simulink model "ChimeIndicatorOutput"  (R2018b)
settings: Solver=FixedStepDiscrete  StartTime=0.0  StopTime=10.0  FixedStep=0.01  RelTol=1e-3
undefined symbols (not defined in the file or in its folder): f, h, IfVeSMSeStNumConfig, KeSMSbMdChime1Enable_Val, KeSMSbSRSPosNumConfig_Val, KeSMSuChmReqDurmTm_Val, KeSMSuChmReqIntlTm_Val, KeSMSwModeChimeReqTm_Val, KeSMSwSRSActiveValidTm_Val, SRSIndicatorStat1
libraries: MSMLib x27
(part 1 of 2)
settings Model: Creator=su3dcu  LastModifiedBy=su3dcu
settings DataIOCC: SaveFormat=StructureWithTime
settings OptimizationCC: DefaultParameterBehavior=Inlined  EnhancedBackFolding=on  PassReuseOutputArgsAs=Individual arguments  ZeroExternalMemoryAtStartup=off  ZeroInternalMemoryAtStartup=off  OptimizeBlockOrder=speed  DifferentSizesBufferReuse=on  OptimizationCustomize=off
settings DebuggingCC: ParameterTunabilityLossMsg=error
settings HardwareCC: ProdBitPerPointer=32  ProdBitPerSizeT=32  ProdBitPerPtrDiffT=32  ProdLargestAtomicFloat=None  ProdWordSize=32  ProdHWDeviceType=Renesas->RH850
settings ModelReferenceCC: ModelReferenceNumInstancesAllowed=Single
settings SFSimCC: MATLABDynamicMemAlloc=off
settings RTWCC: SystemTargetFile=autosar.tlc  GenCodeOnly=on  TemplateMakefile=ert_default_tmf  Description=AUTOSAR  GenerateReport=on  IncludeHyperlinkInReport=on  LaunchReport=on  GenerateTraceInfo=on  GenerateTraceReport=on  GenerateTraceReportSl=on  GenerateTraceReportSf=on  GenerateTraceReportEml=on
settings CodeAppCC: ForceParamTrailComments=on  IgnoreCustomStorageClasses=off  OperatorAnnotations=on  SimulinkDataObjDesc=on  SFDataObjDesc=on  InsertBlockDesc=on
settings STFCustomTargetCC: TargetLangStandard=C99 (ISO)  MultiwordLength=256  ParMdlRefBuildCompliant=on  CompOptLevelCompliant=on  IncludeMdlTerminateFcn=off  CombineOutputUpdateFcns=on  SuppressErrorStatus=on  ERTCustomFileBanners=on  SupportNonFinite=off  SupportComplex=off  SupportContinuousTime=off  SupportNonInlinedSFcns=off  RemoveResetFunc=on  MATLABClassNameForMDSCustomization=Simulink.SoftwareTarget.ERTCustomization  AutosarCompliant=on  UseToolchainInfoCompliant=on  LookupTableObjectStructAxisOrder=2,1,3,4,...  LUTObjectStructOrderEvenSpacing=Size,Table,Breakpoints  SystemTargetFile=autosar.tlc
settings ERTTargetCC: TargetLangStandard=C99 (ISO)  ConcurrentExecutionCompliant=off  IncludeMdlTerminateFcn=off  SuppressErrorStatus=on  SupportNonFinite=off  SupportComplex=off  ModelStepFunctionPrototypeControlCompliant=off  CPPClassGenCompliant=off  AutosarCompliant=on  LookupTableObjectStructAxisOrder=2,1,3,4,...  LUTObjectStructOrderEvenSpacing=Size,Table,Breakpoints  InlinedParameterPlacement=NonHierarchical  ERTCustomFileTemplate=example_file_process.tlc  ERTFilePackagingFormat=Compact

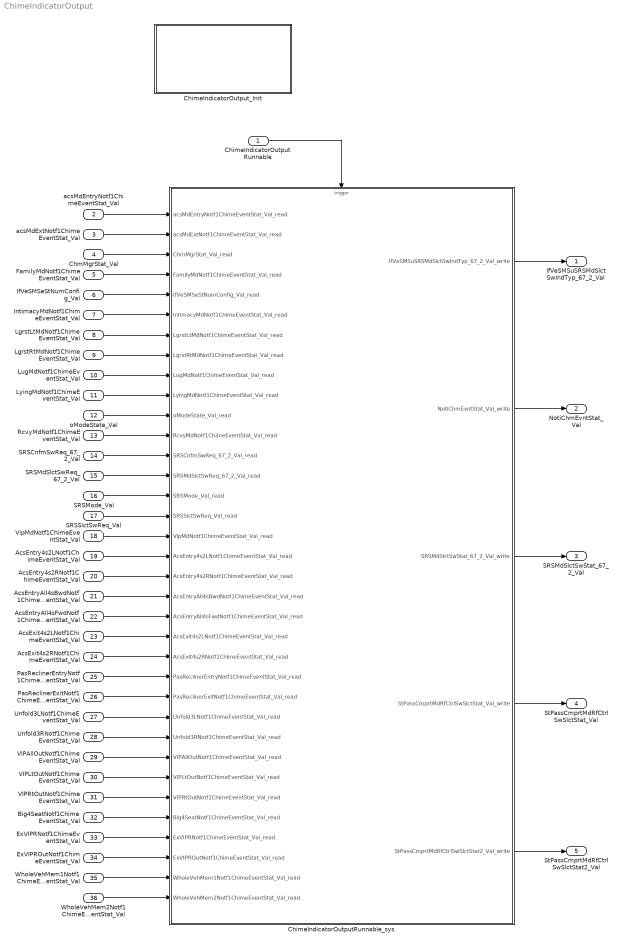
== system ChimeIndicatorOutput ==
  ChimeIndicatorOutputRunnable : Inport  SampleTime=0.01  OutputFunctionCall=on
  acsMdEntryNotf1ChimeEventStat_Val : Inport  Port=2  OutDataTypeStr=boolean  PortDimensions=1
  acsMdExtNotf1ChimeEventStat_Val : Inport  Port=3  OutDataTypeStr=boolean  PortDimensions=1
  ChmMgrStat_Val : Inport  Port=4  OutDataTypeStr=uint16  PortDimensions=1
  FamilyMdNotf1ChimeEventStat_Val : Inport  Port=5  OutDataTypeStr=boolean  PortDimensions=1
  IfVeSMSeStNumConfig_Val : Inport  Port=6  OutDataTypeStr=Enum: IfVeSMSeStNumConfig  PortDimensions=1
  IntimacyMdNotf1ChimeEventStat_Val : Inport  Port=7  OutDataTypeStr=boolean  PortDimensions=1
  LgrstLtMdNotf1ChimeEventStat_Val : Inport  Port=8  OutDataTypeStr=boolean  PortDimensions=1
  LgrstRtMdNotf1ChimeEventStat_Val : Inport  Port=9  OutDataTypeStr=boolean  PortDimensions=1
  LugMdNotf1ChimeEventStat_Val : Inport  Port=10  OutDataTypeStr=boolean  PortDimensions=1
  LyingMdNotf1ChimeEventStat_Val : Inport  Port=11  OutDataTypeStr=boolean  PortDimensions=1
  oModeState_Val : Inport  Port=12  OutDataTypeStr=Enum: MdTp1  PortDimensions=1
  RcvyMdNotf1ChimeEventStat_Val : Inport  Port=13  OutDataTypeStr=boolean  PortDimensions=1
  SRSCnfmSwReq_67_2_Val : Inport  Port=14  OutDataTypeStr=boolean  PortDimensions=1
  SRSMdSlctSwReq_67_2_Val : Inport  Port=15  OutDataTypeStr=Enum: SRSSlctSwStat1  PortDimensions=1
  SRSMode_Val : Inport  Port=16  OutDataTypeStr=Enum: SRSCurMode1  PortDimensions=1
  SRSSlctSwReq_Val : Inport  Port=17  OutDataTypeStr=Enum: SRSMode1  PortDimensions=1
  VipMdNotf1ChimeEventStat_Val : Inport  Port=18  OutDataTypeStr=boolean  PortDimensions=1
  AcsEntry4s2LNotf1ChimeEventStat_Val : Inport  Port=19  OutDataTypeStr=boolean  PortDimensions=1
  AcsEntry4s2RNotf1ChimeEventStat_Val : Inport  Port=20  OutDataTypeStr=boolean  PortDimensions=1
  AcsEntryAll4sBwdNotf1ChimeEventStat_Val : Inport  Port=21  OutDataTypeStr=boolean  PortDimensions=1
  AcsEntryAll4sFwdNotf1ChimeEventStat_Val : Inport  Port=22  OutDataTypeStr=boolean  PortDimensions=1
  AcsExit4s2LNotf1ChimeEventStat_Val : Inport  Port=23  OutDataTypeStr=boolean  PortDimensions=1
  AcsExit4s2RNotf1ChimeEventStat_Val : Inport  Port=24  OutDataTypeStr=boolean  PortDimensions=1
  PasReclinerEntryNotf1ChimeEventStat_Val : Inport  Port=25  OutDataTypeStr=boolean  PortDimensions=1
  PasReclinerExitNotf1ChimeEventStat_Val : Inport  Port=26  OutDataTypeStr=boolean  PortDimensions=1
  Unfold3LNotf1ChimeEventStat_Val : Inport  Port=27  OutDataTypeStr=boolean  PortDimensions=1
  Unfold3RNotf1ChimeEventStat_Val : Inport  Port=28  OutDataTypeStr=boolean  PortDimensions=1
  VIPAllOutNotf1ChimeEventStat_Val : Inport  Port=29  OutDataTypeStr=boolean  PortDimensions=1
  VIPLtOutNotf1ChimeEventStat_Val : Inport  Port=30  OutDataTypeStr=boolean  PortDimensions=1
  VIPRtOutNotf1ChimeEventStat_Val : Inport  Port=31  OutDataTypeStr=boolean  PortDimensions=1
  Big4SeatNotf1ChimeEventStat_Val : Inport  Port=32  OutDataTypeStr=boolean  PortDimensions=1
  ExVIPRNotf1ChimeEventStat_Val : Inport  Port=33  OutDataTypeStr=boolean  PortDimensions=1
  ExVIPROutNotf1ChimeEventStat_Val : Inport  Port=34  OutDataTypeStr=boolean  PortDimensions=1
  WholeVehMem1Notf1ChimeEventStat_Val : Inport  Port=35  OutDataTypeStr=boolean  PortDimensions=1
  WholeVehMem2Notf1ChimeEventStat_Val : Inport  Port=36  OutDataTypeStr=boolean  PortDimensions=1
  ChimeIndicatorOutputRunnable_sys : Subsystem
  ChimeIndicatorOutput_Init : Subsystem
  IfVeSMSuSRSMdSlctSwIndTyp_67_2_Val : Outport  OutDataTypeStr=Enum: SRSSlctSwIndTyp  PortDimensions=1
  NotiChmEvntStat_Val : Outport  Port=2  OutDataTypeStr=Enum: EventSts1  PortDimensions=1
  SRSMdSlctSwStat_67_2_Val : Outport  Port=3  OutDataTypeStr=Enum: SRSIndicatorStat  PortDimensions=1
  StPassCmprtMdRfCtrlSwSlctStat_Val : Outport  Port=4  OutDataTypeStr=Enum: CmprtMdRfCtrlSwSlctStat1  PortDimensions=1
  StPassCmprtMdRfCtrlSwSlctStat2_Val : Outport  Port=5  OutDataTypeStr=Enum: CmprtMdRfCtrlSwSlctStat2  PortDimensions=1
  wires:
  acsMdEntryNotf1ChimeEventStat_Val/1 -> ChimeIndicatorOutputRunnable_sys/1(acsMdEntryNotf1ChimeEventStat_Val_read)
  acsMdExtNotf1ChimeEventStat_Val/1 -> ChimeIndicatorOutputRunnable_sys/2(acsMdExtNotf1ChimeEventStat_Val_read)
  ChmMgrStat_Val/1 -> ChimeIndicatorOutputRunnable_sys/3(ChmMgrStat_Val_read)
  FamilyMdNotf1ChimeEventStat_Val/1 -> ChimeIndicatorOutputRunnable_sys/4(FamilyMdNotf1ChimeEventStat_Val_read)
  IfVeSMSeStNumConfig_Val/1 -> ChimeIndicatorOutputRunnable_sys/5(IfVeSMSeStNumConfig_Val_read)
  IntimacyMdNotf1ChimeEventStat_Val/1 -> ChimeIndicatorOutputRunnable_sys/6(IntimacyMdNotf1ChimeEventStat_Val_read)
  LgrstLtMdNotf1ChimeEventStat_Val/1 -> ChimeIndicatorOutputRunnable_sys/7(LgrstLtMdNotf1ChimeEventStat_Val_read)
  LgrstRtMdNotf1ChimeEventStat_Val/1 -> ChimeIndicatorOutputRunnable_sys/8(LgrstRtMdNotf1ChimeEventStat_Val_read)
  LugMdNotf1ChimeEventStat_Val/1 -> ChimeIndicatorOutputRunnable_sys/9(LugMdNotf1ChimeEventStat_Val_read)
  LyingMdNotf1ChimeEventStat_Val/1 -> ChimeIndicatorOutputRunnable_sys/10(LyingMdNotf1ChimeEventStat_Val_read)
  oModeState_Val/1 -> ChimeIndicatorOutputRunnable_sys/11(oModeState_Val_read)
  RcvyMdNotf1ChimeEventStat_Val/1 -> ChimeIndicatorOutputRunnable_sys/12(RcvyMdNotf1ChimeEventStat_Val_read)
  SRSCnfmSwReq_67_2_Val/1 -> ChimeIndicatorOutputRunnable_sys/13(SRSCnfmSwReq_67_2_Val_read)
  SRSMdSlctSwReq_67_2_Val/1 -> ChimeIndicatorOutputRunnable_sys/14(SRSMdSlctSwReq_67_2_Val_read)
  SRSMode_Val/1 -> ChimeIndicatorOutputRunnable_sys/15(SRSMode_Val_read)
  SRSSlctSwReq_Val/1 -> ChimeIndicatorOutputRunnable_sys/16(SRSSlctSwReq_Val_read)
  VipMdNotf1ChimeEventStat_Val/1 -> ChimeIndicatorOutputRunnable_sys/17(VipMdNotf1ChimeEventStat_Val_read)
  ChimeIndicatorOutputRunnable_sys/1(IfVeSMSuSRSMdSlctSwIndTyp_67_2_Val_write) -> IfVeSMSuSRSMdSlctSwIndTyp_67_2_Val/1
  ChimeIndicatorOutputRunnable_sys/2(NotiChmEvntStat_Val_write) -> NotiChmEvntStat_Val/1
  ChimeIndicatorOutputRunnable_sys/3(SRSMdSlctSwStat_67_2_Val_write) -> SRSMdSlctSwStat_67_2_Val/1
  ChimeIndicatorOutputRunnable_sys/4(StPassCmprtMdRfCtrlSwSlctStat_Val_write) -> StPassCmprtMdRfCtrlSwSlctStat_Val/1
  ChimeIndicatorOutputRunnable_sys/5(StPassCmprtMdRfCtrlSwSlctStat2_Val_write) -> StPassCmprtMdRfCtrlSwSlctStat2_Val/1
  ChimeIndicatorOutputRunnable/1 -> ChimeIndicatorOutputRunnable_sys/Trigger
  AcsEntry4s2LNotf1ChimeEventStat_Val/1 -> ChimeIndicatorOutputRunnable_sys/18(AcsEntry4s2LNotf1ChimeEventStat_Val_read)
  AcsEntry4s2RNotf1ChimeEventStat_Val/1 -> ChimeIndicatorOutputRunnable_sys/19(AcsEntry4s2RNotf1ChimeEventStat_Val_read)
  AcsEntryAll4sBwdNotf1ChimeEventStat_Val/1 -> ChimeIndicatorOutputRunnable_sys/20(AcsEntryAll4sBwdNotf1ChimeEventStat_Val_read)
  AcsEntryAll4sFwdNotf1ChimeEventStat_Val/1 -> ChimeIndicatorOutputRunnable_sys/21(AcsEntryAll4sFwdNotf1ChimeEventStat_Val_read)
  AcsExit4s2LNotf1ChimeEventStat_Val/1 -> ChimeIndicatorOutputRunnable_sys/22(AcsExit4s2LNotf1ChimeEventStat_Val_read)
  AcsExit4s2RNotf1ChimeEventStat_Val/1 -> ChimeIndicatorOutputRunnable_sys/23(AcsExit4s2RNotf1ChimeEventStat_Val_read)
  PasReclinerEntryNotf1ChimeEventStat_Val/1 -> ChimeIndicatorOutputRunnable_sys/24(PasReclinerEntryNotf1ChimeEventStat_Val_read)
  PasReclinerExitNotf1ChimeEventStat_Val/1 -> ChimeIndicatorOutputRunnable_sys/25(PasReclinerExitNotf1ChimeEventStat_Val_read)
  Unfold3LNotf1ChimeEventStat_Val/1 -> ChimeIndicatorOutputRunnable_sys/26(Unfold3LNotf1ChimeEventStat_Val_read)
  Unfold3RNotf1ChimeEventStat_Val/1 -> ChimeIndicatorOutputRunnable_sys/27(Unfold3RNotf1ChimeEventStat_Val_read)
  VIPAllOutNotf1ChimeEventStat_Val/1 -> ChimeIndicatorOutputRunnable_sys/28(VIPAllOutNotf1ChimeEventStat_Val_read)
  VIPLtOutNotf1ChimeEventStat_Val/1 -> ChimeIndicatorOutputRunnable_sys/29(VIPLtOutNotf1ChimeEventStat_Val_read)
  VIPRtOutNotf1ChimeEventStat_Val/1 -> ChimeIndicatorOutputRunnable_sys/30(VIPRtOutNotf1ChimeEventStat_Val_read)
  Big4SeatNotf1ChimeEventStat_Val/1 -> ChimeIndicatorOutputRunnable_sys/31(Big4SeatNotf1ChimeEventStat_Val_read)
  ExVIPRNotf1ChimeEventStat_Val/1 -> ChimeIndicatorOutputRunnable_sys/32(ExVIPRNotf1ChimeEventStat_Val_read)
  ExVIPROutNotf1ChimeEventStat_Val/1 -> ChimeIndicatorOutputRunnable_sys/33(ExVIPROutNotf1ChimeEventStat_Val_read)
  WholeVehMem1Notf1ChimeEventStat_Val/1 -> ChimeIndicatorOutputRunnable_sys/34(WholeVehMem1Notf1ChimeEventStat_Val_read)
  WholeVehMem2Notf1ChimeEventStat_Val/1 -> ChimeIndicatorOutputRunnable_sys/35(WholeVehMem2Notf1ChimeEventStat_Val_read)

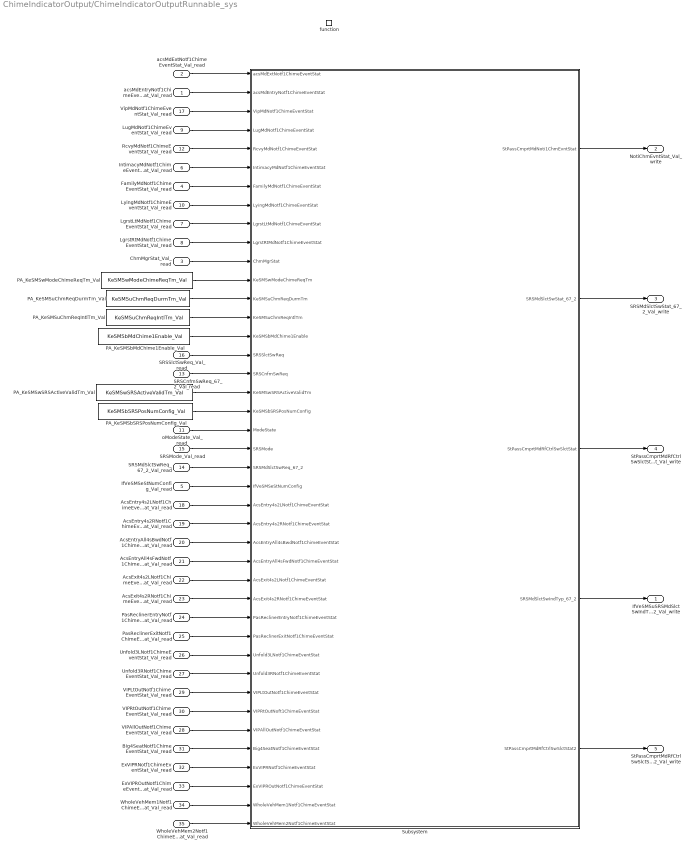
== system ChimeIndicatorOutput/ChimeIndicatorOutputRunnable_sys ==
  acsMdEntryNotf1ChimeEventStat_Val_read : Inport
  acsMdExtNotf1ChimeEventStat_Val_read : Inport  Port=2
  ChmMgrStat_Val_read : Inport  Port=3
  FamilyMdNotf1ChimeEventStat_Val_read : Inport  Port=4
  IfVeSMSeStNumConfig_Val_read : Inport  Port=5
  IntimacyMdNotf1ChimeEventStat_Val_read : Inport  Port=6
  LgrstLtMdNotf1ChimeEventStat_Val_read : Inport  Port=7
  LgrstRtMdNotf1ChimeEventStat_Val_read : Inport  Port=8
  LugMdNotf1ChimeEventStat_Val_read : Inport  Port=9
  LyingMdNotf1ChimeEventStat_Val_read : Inport  Port=10
  oModeState_Val_read : Inport  Port=11
  RcvyMdNotf1ChimeEventStat_Val_read : Inport  Port=12
  SRSCnfmSwReq_67_2_Val_read : Inport  Port=13
  SRSMdSlctSwReq_67_2_Val_read : Inport  Port=14
  SRSMode_Val_read : Inport  Port=15
  SRSSlctSwReq_Val_read : Inport  Port=16
  VipMdNotf1ChimeEventStat_Val_read : Inport  Port=17
  AcsEntry4s2LNotf1ChimeEventStat_Val_read : Inport  Port=18
  AcsEntry4s2RNotf1ChimeEventStat_Val_read : Inport  Port=19
  AcsEntryAll4sBwdNotf1ChimeEventStat_Val_read : Inport  Port=20
  AcsEntryAll4sFwdNotf1ChimeEventStat_Val_read : Inport  Port=21
  AcsExit4s2LNotf1ChimeEventStat_Val_read : Inport  Port=22
  AcsExit4s2RNotf1ChimeEventStat_Val_read : Inport  Port=23
  PasReclinerEntryNotf1ChimeEventStat_Val_read : Inport  Port=24
  PasReclinerExitNotf1ChimeEventStat_Val_read : Inport  Port=25
  Unfold3LNotf1ChimeEventStat_Val_read : Inport  Port=26
  Unfold3RNotf1ChimeEventStat_Val_read : Inport  Port=27
  VIPAllOutNotf1ChimeEventStat_Val_read : Inport  Port=28
  VIPLtOutNotf1ChimeEventStat_Val_read : Inport  Port=29
  VIPRtOutNotf1ChimeEventStat_Val_read : Inport  Port=30
  Big4SeatNotf1ChimeEventStat_Val_read : Inport  Port=31
  ExVIPRNotf1ChimeEventStat_Val_read : Inport  Port=32
  ExVIPROutNotf1ChimeEventStat_Val_read : Inport  Port=33
  WholeVehMem1Notf1ChimeEventStat_Val_read : Inport  Port=34
  WholeVehMem2Notf1ChimeEventStat_Val_read : Inport  Port=35
  function : TriggerPort  TriggerType=function-call  VariantControl=(inherit)  SampleTimeType=periodic  SampleTime=-1
  PA_KeSMSbMdChime1Enable_Val : Constant  Value=KeSMSbMdChime1Enable_Val
  PA_KeSMSbSRSPosNumConfig_Val : Constant  Value=KeSMSbSRSPosNumConfig_Val
  PA_KeSMSuChmReqDurmTm_Val : Constant  Value=KeSMSuChmReqDurmTm_Val
  PA_KeSMSuChmReqIntlTm_Val : Constant  Value=KeSMSuChmReqIntlTm_Val
  PA_KeSMSwModeChimeReqTm_Val : Constant  Value=KeSMSwModeChimeReqTm_Val
  PA_KeSMSwSRSActiveValidTm_Val : Constant  Value=KeSMSwSRSActiveValidTm_Val
  Subsystem : Subsystem
  IfVeSMSuSRSMdSlctSwIndTyp_67_2_Val_write : Outport
  NotiChmEvntStat_Val_write : Outport  Port=2
  SRSMdSlctSwStat_67_2_Val_write : Outport  Port=3
  StPassCmprtMdRfCtrlSwSlctStat_Val_write : Outport  Port=4
  StPassCmprtMdRfCtrlSwSlctStat2_Val_write : Outport  Port=5
  wires:
  acsMdEntryNotf1ChimeEventStat_Val_read/1 -> Subsystem/2(acsMdEntryNotf1ChimeEventStat)
  acsMdExtNotf1ChimeEventStat_Val_read/1 -> Subsystem/1(acsMdExtNotf1ChimeEventStat)
  RcvyMdNotf1ChimeEventStat_Val_read/1 -> Subsystem/5(RcvyMdNotf1ChimeEventStat)
  VipMdNotf1ChimeEventStat_Val_read/1 -> Subsystem/3(VipMdNotf1ChimeEventStat)
  LugMdNotf1ChimeEventStat_Val_read/1 -> Subsystem/4(LugMdNotf1ChimeEventStat)
  IntimacyMdNotf1ChimeEventStat_Val_read/1 -> Subsystem/6(IntimacyMdNotf1ChimeEventStat)
  FamilyMdNotf1ChimeEventStat_Val_read/1 -> Subsystem/7(FamilyMdNotf1ChimeEventStat)
  LyingMdNotf1ChimeEventStat_Val_read/1 -> Subsystem/8(LyingMdNotf1ChimeEventStat)
  LgrstLtMdNotf1ChimeEventStat_Val_read/1 -> Subsystem/9(LgrstLtMdNotf1ChimeEventStat)
  LgrstRtMdNotf1ChimeEventStat_Val_read/1 -> Subsystem/10(LgrstRtMdNotf1ChimeEventStat)
  ChmMgrStat_Val_read/1 -> Subsystem/11(ChmMgrStat)
  oModeState_Val_read/1 -> Subsystem/20(ModeState)
  IfVeSMSeStNumConfig_Val_read/1 -> Subsystem/23(IfVeSMSeStNumConfig)
  SRSMode_Val_read/1 -> Subsystem/21(SRSMode)
  SRSCnfmSwReq_67_2_Val_read/1 -> Subsystem/17(SRSCnfmSwReq)
  PA_KeSMSwModeChimeReqTm_Val/1 -> Subsystem/12(KeSMSwModeChimeReqTm)
  PA_KeSMSuChmReqDurmTm_Val/1 -> Subsystem/13(KeSMSuChmReqDurmTm)
  PA_KeSMSuChmReqIntlTm_Val/1 -> Subsystem/14(KeSMSuChmReqIntlTm)
  PA_KeSMSbMdChime1Enable_Val/1 -> Subsystem/15(KeSMSbMdChime1Enable)
  PA_KeSMSwSRSActiveValidTm_Val/1 -> Subsystem/18(KeSMSwSRSActiveValidTm)
  PA_KeSMSbSRSPosNumConfig_Val/1 -> Subsystem/19(KeSMSbSRSPosNumConfig)
  Subsystem/1(StPassCmprtMdNoti1ChmEvntStat) -> NotiChmEvntStat_Val_write/1
  Subsystem/2(SRSMdSlctSwStat_67_2) -> SRSMdSlctSwStat_67_2_Val_write/1
  Subsystem/3(StPassCmprtMdRfCtrlSwSlctStat) -> StPassCmprtMdRfCtrlSwSlctStat_Val_write/1
  Subsystem/4(SRSMdSlctSwIndTyp_67_2) -> IfVeSMSuSRSMdSlctSwIndTyp_67_2_Val_write/1
  Subsystem/5(StPassCmprtMdRfCtrlSwSlctStat2) -> StPassCmprtMdRfCtrlSwSlctStat2_Val_write/1
  AcsEntry4s2LNotf1ChimeEventStat_Val_read/1 -> Subsystem/24(AcsEntry4s2LNotf1ChimeEventStat)
  AcsEntry4s2RNotf1ChimeEventStat_Val_read/1 -> Subsystem/25(AcsEntry4s2RNotf1ChimeEventStat)
  AcsEntryAll4sBwdNotf1ChimeEventStat_Val_read/1 -> Subsystem/26(AcsEntryAll4sBwdNotf1ChimeEventStat)
  AcsEntryAll4sFwdNotf1ChimeEventStat_Val_read/1 -> Subsystem/27(AcsEntryAll4sFwdNotf1ChimeEventStat)
  AcsExit4s2LNotf1ChimeEventStat_Val_read/1 -> Subsystem/28(AcsExit4s2LNotf1ChimeEventStat)
  AcsExit4s2RNotf1ChimeEventStat_Val_read/1 -> Subsystem/29(AcsExit4s2RNotf1ChimeEventStat)
  SRSMdSlctSwReq_67_2_Val_read/1 -> Subsystem/22(SRSMdSlctSwReq_67_2)
  SRSSlctSwReq_Val_read/1 -> Subsystem/16(SRSSlctSwReq)
  PasReclinerEntryNotf1ChimeEventStat_Val_read/1 -> Subsystem/30(PasReclinerEntryNotf1ChimeEventStat)
  PasReclinerExitNotf1ChimeEventStat_Val_read/1 -> Subsystem/31(PasReclinerExitNotf1ChimeEventStat)
  Unfold3LNotf1ChimeEventStat_Val_read/1 -> Subsystem/32(Unfold3LNotf1ChimeEventStat)
  Unfold3RNotf1ChimeEventStat_Val_read/1 -> Subsystem/33(Unfold3RNotf1ChimeEventStat)
  VIPLtOutNotf1ChimeEventStat_Val_read/1 -> Subsystem/34(VIPLtOutNotf1ChimeEventStat)
  VIPRtOutNotf1ChimeEventStat_Val_read/1 -> Subsystem/35(VIPRtOutNoft1ChimeEventStat)
  VIPAllOutNotf1ChimeEventStat_Val_read/1 -> Subsystem/36(VIPAllOutNotf1ChimeEventStat)
  Big4SeatNotf1ChimeEventStat_Val_read/1 -> Subsystem/37("Big4SeatNotf1ChimeEventStat ")
  ExVIPRNotf1ChimeEventStat_Val_read/1 -> Subsystem/38(ExVIPRNotf1ChimeEventStat)
  ExVIPROutNotf1ChimeEventStat_Val_read/1 -> Subsystem/39(ExVIPROutNotf1ChimeEventStat)
  WholeVehMem1Notf1ChimeEventStat_Val_read/1 -> Subsystem/40(WholeVehMem1Notf1ChimeEventStat)
  WholeVehMem2Notf1ChimeEventStat_Val_read/1 -> Subsystem/41(WholeVehMem2Notf1ChimeEventStat)

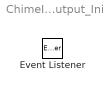
== system ChimeIndicatorOutput/ChimeIndicatorOutput_Init ==
  Event Listener : EventListener  EventName=reset

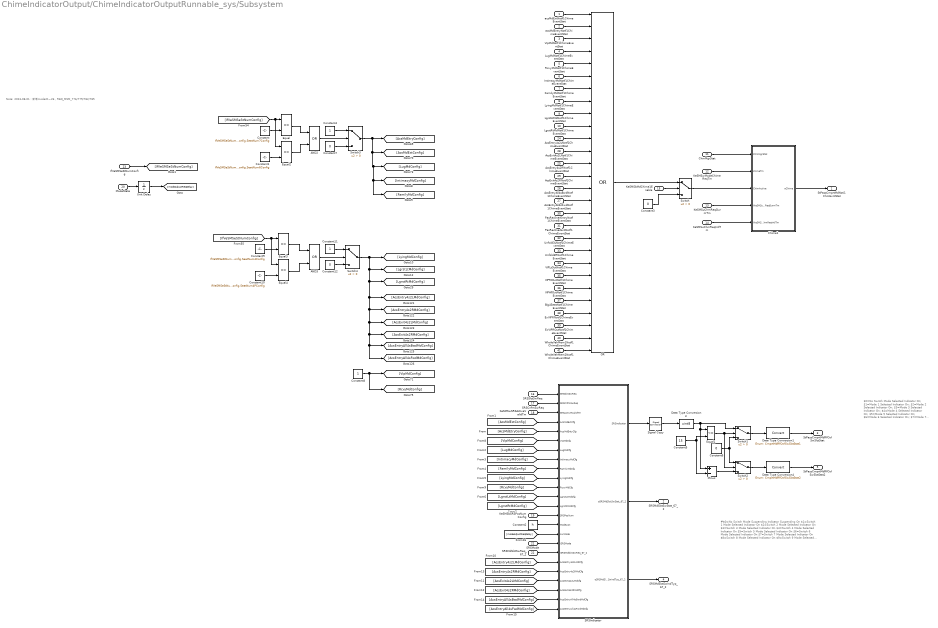
== system ChimeIndicatorOutput/ChimeIndicatorOutputRunnable_sys/Subsystem ==
  note: Note:
      | 2023-08-01：新增mode21~26，REQ_MSM_776/779/782/785
  note: $0=No Switch Mode Selected Indicator On;
      | $1=Mode 1 Selected Indicator On;
      | $2=Mode 2 Selected Indicator On;
      | $3=Mode 3 Selected Indicator On;
      | $4=Mode 4 Selected Indicator On;
      | $5=Mode 5 Selected Indicator On;
      |  $6=Mode 6 Selected Indicator On;
      | $7=Mode 7 Selected Indicator On;
      |  $8=Mode 8 Selected Indicator On;
      |  $9=Mode 9 Selected Indicator On;
      | $A=Mode 10 Selected Indicator On;
      |  $B=Mode 11 Selected Indicator On;
      | $C=Mode 12 Selected Indicator On;
      | $D=Mode 13 Selected Indicator On;
      |  $E=Mode 14 Selected Indicator On;
      | $F=Mode 15 Selected Indicator On
  note: #$0=No Switch Mode Suspending Indicator Suspending On
      | $1=Switch 1 Mode Selected Indicator On
      | $2=Switch 2 Mode Selected Indicator On
      | $3=Switch 3 Mode Selected Indicator On
      | $4=Switch 4 Mode Selected Indicator On
      | $5=Switch 5 Mode Selected Indicator On
      | $6=Switch 6 Mode Selected Indicator On
      | $7=Switch 7 Mode Selected Indicator On
      | $8=Switch 8 Mode Selected Indicator On
      | $9=Switch 9 Mode Selected Indicator On
      | $A=Switch 10 Mode Selected Indicator On
      | $B=Reserved;
      | $C=Reserved;
      | $D=Reserved;
      | $E=Reserved;
      | $F=Reserved;
      | #SRSIndicatorStat和SwitchN Mode Selected Indicator On一一对应
  acsMdExtNotf1ChimeEventStat : Inport
  acsMdEntryNotf1ChimeEventStat : Inport  Port=2
  VipMdNotf1ChimeEventStat : Inport  Port=3
  LugMdNotf1ChimeEventStat : Inport  Port=4
  RcvyMdNotf1ChimeEventStat : Inport  Port=5
  IntimacyMdNotf1ChimeEventStat : Inport  Port=6
  FamilyMdNotf1ChimeEventStat : Inport  Port=7
  LyingMdNotf1ChimeEventStat : Inport  Port=8
  LgrstLtMdNotf1ChimeEventStat : Inport  Port=9
  LgrstRtMdNotf1ChimeEventStat : Inport  Port=10
  ChmMgrStat : Inport  Port=11
  KeSMSwModeChimeReqTm : Inport  Port=12
  KeSMSuChmReqDurmTm : Inport  Port=13
  KeSMSuChmReqIntlTm : Inport  Port=14
  KeSMSbMdChime1Enable : Inport  Port=15
  SRSSlctSwReq : Inport  Port=16
  SRSCnfmSwReq : Inport  Port=17
  KeSMSwSRSActiveValidTm : Inport  Port=18
  KeSMSbSRSPosNumConfig : Inport  Port=19
  ModeState : Inport  Port=20
  SRSMode : Inport  Port=21
  SRSMdSlctSwReq_67_2 : Inport  Port=22
  IfVeSMSeStNumConfig : Inport  Port=23
  AcsEntry4s2LNotf1ChimeEventStat : Inport  Port=24
  AcsEntry4s2RNotf1ChimeEventStat : Inport  Port=25
  AcsEntryAll4sBwdNotf1ChimeEventStat : Inport  Port=26
  AcsEntryAll4sFwdNotf1ChimeEventStat : Inport  Port=27
  AcsExit4s2LNotf1ChimeEventStat : Inport  Port=28
  AcsExit4s2RNotf1ChimeEventStat : Inport  Port=29
  PasReclinerEntryNotf1ChimeEventStat : Inport  Port=30
  PasReclinerExitNotf1ChimeEventStat : Inport  Port=31
  Unfold3LNotf1ChimeEventStat : Inport  Port=32
  Unfold3RNotf1ChimeEventStat : Inport  Port=33
  VIPLtOutNotf1ChimeEventStat : Inport  Port=34
  VIPRtOutNoft1ChimeEventStat : Inport  Port=35
  VIPAllOutNotf1ChimeEventStat : Inport  Port=36
  "Big4SeatNotf1ChimeEventStat " : Inport  Port=37
  ExVIPRNotf1ChimeEventStat : Inport  Port=38
  ExVIPROutNotf1ChimeEventStat : Inport  Port=39
  WholeVehMem1Notf1ChimeEventStat : Inport  Port=40
  WholeVehMem2Notf1ChimeEventStat : Inport  Port=41
  AND2 : Logic  Operator=OR  AllPortsSameDT=off  OutDataTypeStr=boolean
  AND3 : Logic  Operator=OR  AllPortsSameDT=off  OutDataTypeStr=boolean
  Chime1 : Subsystem
  Constant : Constant  Value=IfVeSMSeStNumConfig.SeatNum7Config  OutDataTypeStr=Enum: IfVeSMSeStNumConfig
  Constant1 : Constant  Value=IfVeSMSeStNumConfig.SeatNum6Config  OutDataTypeStr=Enum: IfVeSMSeStNumConfig
  Constant10 : Constant  Value=IfVeSMSeStNumConfig.SeatNum4PConfig  OutDataTypeStr=Enum: IfVeSMSeStNumConfig
  Constant11 : Constant  OutDataTypeStr=boolean
  Constant12 : Constant  Value=0  OutDataTypeStr=boolean
  Constant2 : Constant  Value=h  OutDataTypeStr=uint8
  Constant3 : Constant  Value=0  OutDataTypeStr=boolean
  Constant4 : Constant  OutDataTypeStr=boolean
  Constant5 : Constant  Value=15  OutDataTypeStr=uint8
  Constant6 : Constant  Value=0  OutDataTypeStr=uint8
  Constant7 : Constant  Value=0  OutDataTypeStr=boolean
  Constant8 : Constant  OutDataTypeStr=boolean
  Constant9 : Constant  Value=IfVeSMSeStNumConfig.SeatNum4Config  OutDataTypeStr=Enum: IfVeSMSeStNumConfig
  Data Type Conversion1 : DataTypeConversion  OutDataTypeStr=Enum: CmprtMdRfCtrlSwSlctStat1
  Data Type Conversion3 : DataTypeConversion  OutDataTypeStr=uint8
  Data Type Conversion4 : DataTypeConversion  OutDataTypeStr=Enum: CmprtMdRfCtrlSwSlctStat2
  Equal{,2..4} (4 alike) : RelationalOperator  Operator===  OutDataTypeStr=boolean  RndMeth=Simplest
  Equal1 : RelationalOperator  Operator=<=  OutDataTypeStr=boolean  RndMeth=Simplest
  Minus : Sum  Inputs=+-
  OR : Logic  Operator=OR  Inputs=28  AllPortsSameDT=off  OutDataTypeStr=boolean
  SRSIndicator : Subsystem
  Signal Copy : SignalConversion  OverrideOpt=off
  Switch{,1..4} (5 alike) : Switch  Criteria=u2 > Threshold
  Unit Delay : UnitDelay  InitialCondition=f  SampleTime=-1
  StPassCmprtMdNoti1ChmEvntStat : Outport  VectorParamsAs1DForOutWhenUnconnected=on
  SRSMdSlctSwStat_67_2 : Outport  Port=2
  StPassCmprtMdRfCtrlSwSlctStat : Outport  Port=3
  SRSMdSlctSwIndTyp_67_2 : Outport  Port=4
  StPassCmprtMdRfCtrlSwSlctStat2 : Outport  Port=5
  wires:
  LyingMdNotf1ChimeEventStat/1 -> OR/8
  ChmMgrStat/1 -> Chime1/1(ChmMgrStat)
  KeSMSuChmReqIntlTm/1 -> Chime1/5(iKeSMSuChmReqIntlTm)
  FamilyMdNotf1ChimeEventStat/1 -> OR/7
  LgrstLtMdNotf1ChimeEventStat/1 -> OR/9
  KeSMSuChmReqDurmTm/1 -> Chime1/4(iKeSMSuChmReqDurmTm)
  VipMdNotf1ChimeEventStat/1 -> OR/3
  KeSMSbMdChime1Enable/1 -> Switch/2
  LgrstRtMdNotf1ChimeEventStat/1 -> OR/10
  IntimacyMdNotf1ChimeEventStat/1 -> OR/6
  OR/1 -> Switch/1
  KeSMSwModeChimeReqTm/1 -> Chime1/2(chimeTm)
  acsMdExtNotf1ChimeEventStat/1 -> OR/1
  RcvyMdNotf1ChimeEventStat/1 -> OR/5
  acsMdEntryNotf1ChimeEventStat/1 -> OR/2
  LugMdNotf1ChimeEventStat/1 -> OR/4
  Chime1/1(oChime) -> StPassCmprtMdNoti1ChmEvntStat/1
  Constant3/1 -> Switch/3
  Switch/1 -> Chime1/3(ChimActive)
  SRSMdSlctSwReq_67_2/1 -> SRSIndicator/18(iSRSMdSlctSwReq_67_2)
  Data Type Conversion1/1 -> StPassCmprtMdRfCtrlSwSlctStat/1
  Switch1/1 -> Data Type Conversion1/1
  Data Type Conversion4/1 -> StPassCmprtMdRfCtrlSwSlctStat2/1
  Switch2/1 -> Data Type Conversion4/1
  Constant6/1 -> Switch2/1, Switch1/3
  Minus/1 -> Switch2/3
  Equal1/1 -> Switch2/2, Switch1/2
  SRSIndicator/2(oSRSMdSlctSwStat_67_2) -> SRSMdSlctSwStat_67_2/1
  Constant2/1 -> SRSIndicator/15("ModeList ")
  KeSMSbSRSPosNumConfig/1 -> SRSIndicator/14(SRSPosNum)
  Data Type Conversion3/1 -> Switch1/1, Minus/1, Equal1/1
  Signal Copy/1 -> Data Type Conversion3/1
  SRSSlctSwReq/1 -> SRSIndicator/1(SRSSlctSwReq)
  KeSMSwSRSActiveValidTm/1 -> SRSIndicator/3(SRSActiveValidTm)
  SRSIndicator/3(oSRSMdSlctSwIndTyp_67_2) -> SRSMdSlctSwIndTyp_67_2/1
  SRSMode/1 -> SRSIndicator/17("iSRSMode ")
  Constant5/1 -> Minus/2, Equal1/2
  SRSIndicator/1(SRSIndicator) -> Signal Copy/1
  SRSCnfmSwReq/1 -> SRSIndicator/2(SRSCnfmSwReq)
  ModeState/1 -> Unit Delay/1
  Unit Delay/1 -> [modeAdjustReqDelay]
  Equal/1 -> AND2/1
  Constant1/1 -> Equal2/2
  Switch4/1 -> [AcsEntryAll4sFwdMdConfig], [AcsEntryAll4sBwdMdConfig], [AcsExit4s2RMdConfig], [AcsExit4s2LMdConfig], [AcsEntry4s2RMdConfig], [AcsEntry4s2LMdConfig], [LgrstRtMdConfig], [LgrstLtMdConfig], [LyingMdConfig]
  Constant10/1 -> Equal4/2
  Constant9/1 -> Equal3/2
  [IfVeSMSeStNumConfig] -> Equal4/1, Equal3/1
  Constant11/1 -> Switch4/1
  Constant12/1 -> Switch4/3
  AND3/1 -> Switch4/2
  Constant4/1 -> Switch3/1
  Constant7/1 -> Switch3/3
  Equal4/1 -> AND3/2
  Constant8/1 -> [RcvyMdConfig], [VipMdConfig]
  Equal2/1 -> AND2/2
  [IfVeSMSeStNumConfig] -> Equal2/1, Equal/1
  Equal3/1 -> AND3/1
  Constant/1 -> Equal/2
  Switch3/1 -> [FamilyMdConfig], [IntimacyMdConfig], [LugMdConfig], [AcsMdExtConfig], [AcsMdEtryConfig]
  AND2/1 -> Switch3/2
  IfVeSMSeStNumConfig/1 -> [IfVeSMSeStNumConfig]
  [AcsMdEtryConfig] -> SRSIndicator/5(AcsMdEntyCfg)
  [AcsMdExtConfig] -> SRSIndicator/4(AcsMdExtCfg)
  [LugMdConfig] -> SRSIndicator/7(LugMdCfg)
  [IntimacyMdConfig] -> SRSIndicator/8(IntimacyMdCfg)
  [FamilyMdConfig] -> SRSIndicator/9(FamilyMdCfg)
  [LyingMdConfig] -> SRSIndicator/10(LyingMdCfg)
  [LgrstLtMdConfig] -> SRSIndicator/12(LgrstLtMdCfg)
  [LgrstRtMdConfig] -> SRSIndicator/13(LgrstRtMdCfg)
  [VipMdConfig] -> SRSIndicator/6(VipMdCfg)
  [RcvyMdConfig] -> SRSIndicator/11(RcvyMdCfg)
  [AcsEntry4s2LMdConfig] -> SRSIndicator/19(AcsEntry4s2LMdCfg)
  [AcsEntry4s2RMdConfig] -> SRSIndicator/20(AcsEntry4s2RMdCfg)
  [AcsExit4s2LMdConfig] -> SRSIndicator/21(AcsExit4s2LMdCfg)
  [AcsExit4s2RMdConfig] -> SRSIndicator/22(AcsExit4s2RMdCfg)
  [AcsEntryAll4sBwdMdConfig] -> SRSIndicator/23(AcsEntryAll4sBwdMdCfg)
  [AcsEntryAll4sFwdMdConfig] -> SRSIndicator/24(AcsEntryAll4sFwdMdCfg)
  AcsEntry4s2LNotf1ChimeEventStat/1 -> OR/11
  AcsExit4s2LNotf1ChimeEventStat/1 -> OR/12
  AcsEntry4s2RNotf1ChimeEventStat/1 -> OR/13
  AcsExit4s2RNotf1ChimeEventStat/1 -> OR/14
  AcsEntryAll4sBwdNotf1ChimeEventStat/1 -> OR/15
  AcsEntryAll4sFwdNotf1ChimeEventStat/1 -> OR/16
  PasReclinerEntryNotf1ChimeEventStat/1 -> OR/17
  PasReclinerExitNotf1ChimeEventStat/1 -> OR/18
  Unfold3LNotf1ChimeEventStat/1 -> OR/19
  Unfold3RNotf1ChimeEventStat/1 -> OR/20
  VIPLtOutNotf1ChimeEventStat/1 -> OR/21
  VIPRtOutNoft1ChimeEventStat/1 -> OR/22
  VIPAllOutNotf1ChimeEventStat/1 -> OR/23
  [modeAdjustReqDelay] -> SRSIndicator/16(curMode)
  "Big4SeatNotf1ChimeEventStat "/1 -> OR/24
  ExVIPRNotf1ChimeEventStat/1 -> OR/25
  ExVIPROutNotf1ChimeEventStat/1 -> OR/26
  WholeVehMem1Notf1ChimeEventStat/1 -> OR/27
  WholeVehMem2Notf1ChimeEventStat/1 -> OR/28

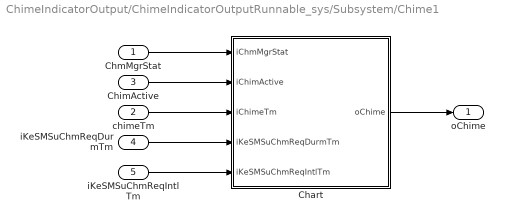
== system ChimeIndicatorOutput/ChimeIndicatorOutputRunnable_sys/Subsystem/Chime1 ==
  ChmMgrStat : Inport
  chimeTm : Inport  Port=2
  ChimActive : Inport  Port=3
  iKeSMSuChmReqDurmTm : Inport  Port=4
  iKeSMSuChmReqIntlTm : Inport  Port=5
  Chart : Stateflow chart  TreatAsAtomicUnit=on
  oChime : Outport
  wires:
  chimeTm/1 -> Chart/3(iChimeTm)
  Chart/1(oChime) -> oChime/1
  ChmMgrStat/1 -> Chart/1(iChmMgrStat)
  ChimActive/1 -> Chart/2(iChimActive)
  iKeSMSuChmReqDurmTm/1 -> Chart/4(iKeSMSuChmReqDurmTm)
  iKeSMSuChmReqIntlTm/1 -> Chart/5(iKeSMSuChmReqIntlTm)

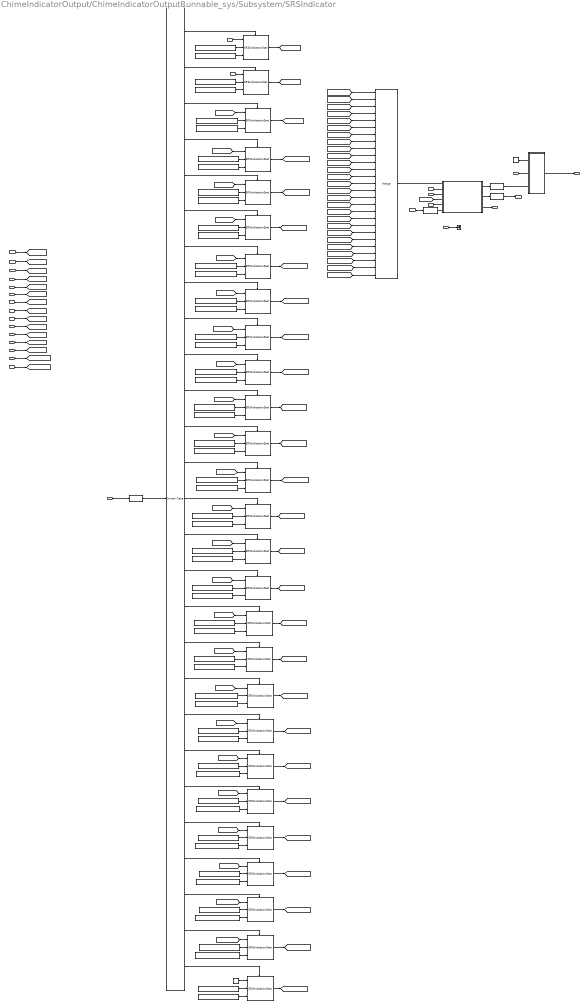
== system ChimeIndicatorOutput/ChimeIndicatorOutputRunnable_sys/Subsystem/SRSIndicator ==
  SRSSlctSwReq : Inport
  SRSCnfmSwReq : Inport  Port=2
  SRSActiveValidTm : Inport  Port=3
  AcsMdExtCfg : Inport  Port=4
  AcsMdEntyCfg : Inport  Port=5
  VipMdCfg : Inport  Port=6
  LugMdCfg : Inport  Port=7
  IntimacyMdCfg : Inport  Port=8
  FamilyMdCfg : Inport  Port=9
  LyingMdCfg : Inport  Port=10
  RcvyMdCfg : Inport  Port=11
  LgrstLtMdCfg : Inport  Port=12
  LgrstRtMdCfg : Inport  Port=13
  SRSPosNum : Inport  Port=14
  "ModeList " : Inport  Port=15
  curMode : Inport  Port=16
  "iSRSMode " : Inport  Port=17
  iSRSMdSlctSwReq_67_2 : Inport  Port=18
  AcsEntry4s2LMdCfg : Inport  Port=19
  AcsEntry4s2RMdCfg : Inport  Port=20
  AcsExit4s2LMdCfg : Inport  Port=21
  AcsExit4s2RMdCfg : Inport  Port=22
  AcsEntryAll4sBwdMdCfg : Inport  Port=23
  AcsEntryAll4sFwdMdCfg : Inport  Port=24
  Chart : Stateflow chart  TreatAsAtomicUnit=on
  Constant : Constant  Value=true  OutDataTypeStr=boolean
  Constant1 : Constant  Value=SRSIndicatorStat1.SRSIndicatorStat1_EzeExit  OutDataTypeStr=Enum:SRSIndicatorStat1
  Constant{2,4,6,8,10..11,13,15,17,19,21,23,25,27,29,31,33..34,36,38,40,42,44,46,48,50,52,54} (28 alike) : Constant  Value=SRSIndicatorStat1.SRSIndicatorStat1_NoIndicator  OutDataTypeStr=Enum:SRSIndicatorStat1
  Constant12 : Constant  Value=SRSIndicatorStat1.SRSIndicatorStat1_RtLug  OutDataTypeStr=Enum:SRSIndicatorStat1
  Constant14 : Constant  Value=SRSIndicatorStat1.SRSIndicatorStat1_AllLug  OutDataTypeStr=Enum:SRSIndicatorStat1
  Constant16 : Constant  Value=26  OutDataTypeStr=uint8
  Constant18 : Constant  Value=SRSIndicatorStat1.SRSIndicatorStat1_IntimacyL  OutDataTypeStr=Enum:SRSIndicatorStat1
  Constant20 : Constant  Value=SRSIndicatorStat1.SRSIndicatorStat1_FamilyR  OutDataTypeStr=Enum:SRSIndicatorStat1
  Constant22 : Constant  Value=SRSIndicatorStat1.SRSIndicatorStat1_FamilyL  OutDataTypeStr=Enum:SRSIndicatorStat1
  Constant24 : Constant  Value=SRSIndicatorStat1.SRSIndicatorStat1_EzeEntry  OutDataTypeStr=Enum:SRSIndicatorStat1
  Constant26 : Constant  Value=SRSIndicatorStat1.SRSIndicatorStat1_RcvyL  OutDataTypeStr=Enum:SRSIndicatorStat1
  Constant28 : Constant  Value=SRSIndicatorStat1.SRSIndicatorStat1_RcvyR  OutDataTypeStr=Enum:SRSIndicatorStat1
  Constant3 : Constant  Value=SRSIndicatorStat1.SRSIndicatorStat1_LfVip  OutDataTypeStr=Enum:SRSIndicatorStat1
  Constant30 : Constant  Value=SRSIndicatorStat1.SRSIndicatorStat1_LyingL  OutDataTypeStr=Enum:SRSIndicatorStat1
  Constant32 : Constant  Value=SRSIndicatorStat1.SRSIndicatorStat1_LyingR  OutDataTypeStr=Enum:SRSIndicatorStat1
  Constant35 : Constant  Value=SRSIndicatorStat1.SRSIndicatorStat1_LgrstOpenLt  OutDataTypeStr=Enum:SRSIndicatorStat1
  Constant37 : Constant  Value=SRSIndicatorStat1.SRSIndicatorStat1_LgrstCloseLt  OutDataTypeStr=Enum:SRSIndicatorStat1
  Constant39 : Constant  Value=SRSIndicatorStat1.SRSIndicatorStat1_LgrstOpenRt  OutDataTypeStr=Enum:SRSIndicatorStat1
  Constant41 : Constant  Value=SRSIndicatorStat1.SRSIndicatorStat1_LgrstCloseRt  OutDataTypeStr=Enum:SRSIndicatorStat1
  Constant43 : Constant  Value=SRSIndicatorStat1.SRSIndicatorStat1_IntimacyR  OutDataTypeStr=Enum:SRSIndicatorStat1
  Constant45 : Constant  Value=SRSIndicatorStat1.SRSIndicatorStat1_EzeEntry4s2L  OutDataTypeStr=Enum:SRSIndicatorStat1
  Constant47 : Constant  Value=SRSIndicatorStat1.SRSIndicatorStat1_EzeExt4s2L  OutDataTypeStr=Enum:SRSIndicatorStat1
  Constant49 : Constant  Value=SRSIndicatorStat1.SRSIndicatorStat1_EzeEntry4s2R  OutDataTypeStr=Enum:SRSIndicatorStat1
  Constant5 : Constant  Value=SRSIndicatorStat1.SRSIndicatorStat1_RtVip  OutDataTypeStr=Enum:SRSIndicatorStat1
  Constant51 : Constant  Value=SRSIndicatorStat1.SRSIndicatorStat1_EzeExt4s2R  OutDataTypeStr=Enum:SRSIndicatorStat1
  Constant53 : Constant  Value=SRSIndicatorStat1.SRSIndicatorStat1_EzeEntryAll4sBwd  OutDataTypeStr=Enum:SRSIndicatorStat1
  Constant55 : Constant  Value=SRSIndicatorStat1.SRSIndicatorStat1_EzeEntryAll4sFwd  OutDataTypeStr=Enum:SRSIndicatorStat1
  Constant7 : Constant  Value=SRSIndicatorStat1.SRSIndicatorStat1_AllVip  OutDataTypeStr=Enum:SRSIndicatorStat1
  Constant9 : Constant  Value=SRSIndicatorStat1.SRSIndicatorStat1_LfLug  OutDataTypeStr=Enum:SRSIndicatorStat1
  Data Type Conversion : DataTypeConversion  OutDataTypeStr=uint8
  Data Type Conversion1 : DataTypeConversion  OutDataTypeStr=uint8
  Data Type Conversion2 : DataTypeConversion  OutDataTypeStr=uint8
  Data Type Conversion4 : DataTypeConversion  OutDataTypeStr=Enum: SRSIndicatorStat
  Merge : Merge  Inputs=27
  SRSIndicationStat {,1..26} (27 alike) : MSMLib/SRSIndicationStat   SystemSampleTime=-1
  Subsystem : Subsystem
  Switch Case : SwitchCase  CaseConditions={1,2,3,4,5,6,7,8,9,10,11,12,13,14,15,16,17,18,19,20,21,22,23,24,25,26}
  Terminator2 : Terminator
  SRSIndicator : Outport
  oSRSMdSlctSwStat_67_2 : Outport  Port=2
  oSRSMdSlctSwIndTyp_67_2 : Outport  Port=3
  wires:
  AcsMdExtCfg/1 -> SRSIndicationStat 1/1
  Switch Case/2 -> SRSIndicationStat 1/Action
  Switch Case/5 -> SRSIndicationStat 4/Action
  Switch Case/6 -> SRSIndicationStat 5/Action
  Switch Case/7 -> SRSIndicationStat 6/Action
  Switch Case/8 -> SRSIndicationStat 7/Action
  Switch Case/27 -> SRSIndicationStat 15/Action
  SRSSlctSwReq/1 -> Data Type Conversion/1
  Data Type Conversion/1 -> Switch Case/1
  SRSCnfmSwReq/1 -> Chart/2(iIsActive)
  SRSActiveValidTm/1 -> Chart/3(iValideTm)
  SRSIndicationStat 5/1 -> [LtLugIndStat]
  [AcsEntyIndStat] -> Merge/1
  [AcsExtIndStat] -> Merge/2
  [LfVipIndStat] -> Merge/3
  [RtVipIndStat] -> Merge/4
  [AllVipIndStat] -> Merge/5
  [LtLugIndStat] -> Merge/6
  [RtLugIndStat] -> Merge/7
  [AllLugIndStat] -> Merge/8
  LugMdCfg/1 -> [LugMdCfg]
  VipMdCfg/1 -> [VipMdCfg]
  FamilyMdCfg/1 -> [FamilyMdCfg]
  LyingMdCfg/1 -> [LyingMdCfg]
  Constant25/1 -> "SRSIndicationStat "/2
  Constant24/1 -> "SRSIndicationStat "/3
  AcsMdEntyCfg/1 -> "SRSIndicationStat "/1
  "SRSIndicationStat "/1 -> [AcsEntyIndStat]
  SRSIndicationStat 1/1 -> [AcsExtIndStat]
  Constant2/1 -> SRSIndicationStat 1/2
  Constant1/1 -> SRSIndicationStat 1/3
  Switch Case/3 -> SRSIndicationStat 2/Action
  [VipMdCfg] -> SRSIndicationStat 2/1
  Constant4/1 -> SRSIndicationStat 2/2
  Constant3/1 -> SRSIndicationStat 2/3
  SRSIndicationStat 2/1 -> [LfVipIndStat]
  [VipMdCfg] -> SRSIndicationStat 3/1
  Constant6/1 -> SRSIndicationStat 3/2
  Constant5/1 -> SRSIndicationStat 3/3
  SRSIndicationStat 3/1 -> [RtVipIndStat]
  [VipMdCfg] -> SRSIndicationStat 4/1
  Constant7/1 -> SRSIndicationStat 4/3
  Constant8/1 -> SRSIndicationStat 4/2
  SRSIndicationStat 4/1 -> [AllVipIndStat]
  Switch Case/4 -> SRSIndicationStat 3/Action
  [LugMdCfg] -> SRSIndicationStat 5/1
  Constant10/1 -> SRSIndicationStat 5/2
  Constant9/1 -> SRSIndicationStat 5/3
  SRSIndicationStat 6/1 -> [RtLugIndStat]
  [LugMdCfg] -> SRSIndicationStat 6/1
  Constant11/1 -> SRSIndicationStat 6/2
  Constant12/1 -> SRSIndicationStat 6/3
  SRSIndicationStat 7/1 -> [AllLugIndStat]
  [LugMdCfg] -> SRSIndicationStat 7/1
  Constant13/1 -> SRSIndicationStat 7/2
  Constant14/1 -> SRSIndicationStat 7/3
  Switch Case/9 -> SRSIndicationStat 8/Action
  Constant17/1 -> SRSIndicationStat 8/2
  Constant18/1 -> SRSIndicationStat 8/3
  SRSIndicationStat 8/1 -> [IntimacyLIndStat]
  Switch Case/10 -> SRSIndicationStat 9/Action
  SRSIndicationStat 9/1 -> [FamiLyRIndStat]
  [FamilyMdCfg] -> SRSIndicationStat 9/1
  Constant19/1 -> SRSIndicationStat 9/2
  Constant20/1 -> SRSIndicationStat 9/3
  Switch Case/11 -> SRSIndicationStat 10/Action
  [FamilyMdCfg] -> SRSIndicationStat 10/1
  Constant21/1 -> SRSIndicationStat 10/2
  Constant22/1 -> SRSIndicationStat 10/3
  SRSIndicationStat 10/1 -> [FamiLyLIndStat]
  Switch Case/12 -> SRSIndicationStat 11/Action
  RcvyMdCfg/1 -> [RcvyMdCfg]
  [RcvyMdCfg] -> SRSIndicationStat 11/1
  Constant23/1 -> SRSIndicationStat 11/2
  Constant26/1 -> SRSIndicationStat 11/3
  SRSIndicationStat 11/1 -> [RcvyLIndStat]
  Switch Case/13 -> SRSIndicationStat 12/Action
  [RcvyMdCfg] -> SRSIndicationStat 12/1
  Constant27/1 -> SRSIndicationStat 12/2
  Constant28/1 -> SRSIndicationStat 12/3
  SRSIndicationStat 12/1 -> [RcvyRIndStat]
  Switch Case/14 -> SRSIndicationStat 13/Action
  SRSIndicationStat 13/1 -> [LyingLIndStat]
  [LyingMdCfg] -> SRSIndicationStat 13/1
  Constant29/1 -> SRSIndicationStat 13/2
  Constant30/1 -> SRSIndicationStat 13/3
  Switch Case/15 -> SRSIndicationStat 14/Action
  [LyingMdCfg] -> SRSIndicationStat 14/1
  Constant31/1 -> SRSIndicationStat 14/2
  Constant32/1 -> SRSIndicationStat 14/3
  SRSIndicationStat 14/1 -> [LyingRIndStat]
  Constant/1 -> SRSIndicationStat 15/1
  Constant15/1 -> SRSIndicationStat 15/2
  Constant33/1 -> SRSIndicationStat 15/3
  SRSIndicationStat 15/1 -> [DefaultIndStat]
  [IntimacyLIndStat] -> Merge/9
  [FamiLyRIndStat] -> Merge/10
  [FamiLyLIndStat] -> Merge/11
  [RcvyLIndStat] -> Merge/12
  [RcvyRIndStat] -> Merge/13
  [LyingLIndStat] -> Merge/14
  [LyingRIndStat] -> Merge/15
  Merge/1 -> Chart/1(iSlctSwStat)
  Chart/1(oSRSIndicatorStat) -> Data Type Conversion2/1
  SRSPosNum/1 -> Terminator2/1
  Data Type Conversion2/1 -> Subsystem/3(data)
  Subsystem/1("index ") -> SRSIndicator/1
  "ModeList "/1 -> Subsystem/2(PosArray)
  Constant16/1 -> Subsystem/1(len)
  [curMode] -> Chart/4(icurMode)
  curMode/1 -> [curMode]
  "iSRSMode "/1 -> Chart/5(iSRSMode)
  LgrstLtMdCfg/1 -> [LgrstLtMdCfg]
  LgrstRtMdCfg/1 -> [LgrstRtMdCfg]
  Switch Case/1 -> "SRSIndicationStat "/Action
  Constant34/1 -> SRSIndicationStat 16/2
  Constant35/1 -> SRSIndicationStat 16/3
  SRSIndicationStat 16/1 -> [LgrstOpenLtIndStat]
  [LgrstLtMdCfg] -> SRSIndicationStat 16/1
  Switch Case/16 -> SRSIndicationStat 16/Action
  Constant37/1 -> SRSIndicationStat 17/3
  SRSIndicationStat 17/1 -> [LgrstCloseLtIndStat]
  Constant36/1 -> SRSIndicationStat 17/2
  Switch Case/17 -> SRSIndicationStat 17/Action
  [LgrstLtMdCfg] -> SRSIndicationStat 17/1
  [LgrstRtMdCfg] -> SRSIndicationStat 18/1
  Constant39/1 -> SRSIndicationStat 18/3
  SRSIndicationStat 18/1 -> [LgrstOpenRtIndStat]
  Constant38/1 -> SRSIndicationStat 18/2
  Switch Case/18 -> SRSIndicationStat 18/Action
  Constant41/1 -> SRSIndicationStat 19/3
  [LgrstRtMdCfg] -> SRSIndicationStat 19/1
  SRSIndicationStat 19/1 -> [LgrstCloseRtIndStat]
  Constant40/1 -> SRSIndicationStat 19/2
  Switch Case/19 -> SRSIndicationStat 19/Action
  [LgrstOpenLtIndStat] -> Merge/16
  [LgrstCloseLtIndStat] -> Merge/17
  [LgrstOpenRtIndStat] -> Merge/18
  [LgrstCloseRtIndStat] -> Merge/19
  IntimacyMdCfg/1 -> [IntimacyMdCfg]
  [IntimacyMdCfg] -> SRSIndicationStat 8/1
  Constant43/1 -> SRSIndicationStat 20/3
  SRSIndicationStat 20/1 -> [IntimacyRIndStat]
  [IntimacyMdCfg] -> SRSIndicationStat 20/1
  Constant42/1 -> SRSIndicationStat 20/2
  Switch Case/20 -> SRSIndicationStat 20/Action
  [IntimacyRIndStat] -> Merge/20
  Data Type Conversion1/1 -> Chart/6(iSRSMdSlctSwReq_67_2)
  iSRSMdSlctSwReq_67_2/1 -> Data Type Conversion1/1
  Chart/2(oSRSMdSlctSwStat) -> Data Type Conversion4/1
  Data Type Conversion4/1 -> oSRSMdSlctSwStat_67_2/1
  Chart/3(oSRSMdSlctSwIndTyp) -> oSRSMdSlctSwIndTyp_67_2/1
  AcsEntry4s2LMdCfg/1 -> [AcsEntry4s2LMdCfg]
  AcsExit4s2LMdCfg/1 -> [AcsExit4s2LMdCfg]
  AcsExit4s2RMdCfg/1 -> [AcsExit4s2RMdCfg]
  AcsEntry4s2RMdCfg/1 -> [AcsEntry4s2RMdCfg]
  AcsEntryAll4sBwdMdCfg/1 -> [AcsEntryAll4sBwdMdCfg]
  AcsEntryAll4sFwdMdCfg/1 -> [AcsEntryAll4sFwdMdCfg]
  Switch Case/21 -> SRSIndicationStat 21/Action
  [AcsEntry4s2LMdCfg] -> SRSIndicationStat 21/1
  Constant44/1 -> SRSIndicationStat 21/2
  Constant45/1 -> SRSIndicationStat 21/3
  SRSIndicationStat 21/1 -> [EzeEntry4s2LIndStat]
  [AcsExit4s2LMdCfg] -> SRSIndicationStat 22/1
  Switch Case/22 -> SRSIndicationStat 22/Action
  Constant46/1 -> SRSIndicationStat 22/2
  Constant47/1 -> SRSIndicationStat 22/3
  SRSIndicationStat 22/1 -> [EzeExt4s2LIndStat]
  [AcsEntry4s2RMdCfg] -> SRSIndicationStat 23/1
  Constant48/1 -> SRSIndicationStat 23/2
  Constant49/1 -> SRSIndicationStat 23/3
  SRSIndicationStat 23/1 -> [EzeEntry4s2RIndStat]
  Switch Case/23 -> SRSIndicationStat 23/Action
  [AcsExit4s2RMdCfg] -> SRSIndicationStat 24/1
  Switch Case/24 -> SRSIndicationStat 24/Action
  Constant50/1 -> SRSIndicationStat 24/2
  Constant51/1 -> SRSIndicationStat 24/3
  SRSIndicationStat 24/1 -> [EzeExt4s2RIndStat]
  Switch Case/25 -> SRSIndicationStat 25/Action
  [AcsEntryAll4sBwdMdCfg] -> SRSIndicationStat 25/1
  Constant52/1 -> SRSIndicationStat 25/2
  Constant53/1 -> SRSIndicationStat 25/3
  SRSIndicationStat 25/1 -> [EzeEntryAll4sBwdIndStat]
  Switch Case/26 -> SRSIndicationStat 26/Action
  [AcsEntryAll4sFwdMdCfg] -> SRSIndicationStat 26/1
  Constant54/1 -> SRSIndicationStat 26/2
  Constant55/1 -> SRSIndicationStat 26/3
  SRSIndicationStat 26/1 -> [EzeEntryAll4sFwdIndStat]
  [EzeEntry4s2LIndStat] -> Merge/21
  [EzeExt4s2LIndStat] -> Merge/22
  [EzeEntry4s2RIndStat] -> Merge/23
  [EzeExt4s2RIndStat] -> Merge/24
  [EzeEntryAll4sBwdIndStat] -> Merge/25
  [EzeEntryAll4sFwdIndStat] -> Merge/26
  [DefaultIndStat] -> Merge/27

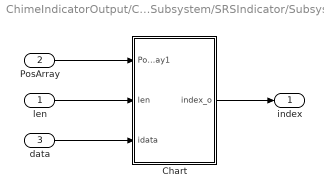
== system ChimeIndicatorOutput/ChimeIndicatorOutputRunnable_sys/Subsystem/SRSIndicator/Subsystem ==
  len : Inport
  PosArray : Inport  Port=2
  data : Inport  Port=3
  Chart : Stateflow chart  TreatAsAtomicUnit=on
  "index " : Outport
  wires:
  PosArray/1 -> Chart/1(PosArray1)
  Chart/1(index_o) -> "index "/1
  len/1 -> Chart/2(len)
  data/1 -> Chart/3(idata)

== stateflow chart ChimeIndicatorOutput/ChimeIndicatorOutputRunnable_sys/Subsystem/Chime1/Chart ==
  state Init
    en:
    ChmReqDurmCnt = (iKeSMSuChmReqDurmTm/10+1);
    ChmReqIntlCnt = (iKeSMSuChmReqIntlTm/10-1);
  state CheckStat
    state Idle
      en:
      oChime = EventSts1.EventSts_NoAct;
    state Active
      state ActiveStage1
        en:
        oChime = EventSts1.EventSts_NoAct;
        tickCount = 0;
        du:
        oChime = EventSts1.EventSts_Act;
      state SendAgain
        en:
        iSendCout = 0;
        tickCount++;
        du:
        tickCount++;
      state ActiveStage2
        en:
        oChime = EventSts1.EventSts_NoAct;
        iSendCout++;
        tickCount++;
        du:
        tickCount++;
      state Idle
      (default) -> ActiveStage1
      CheckStat.Active.Idle -> ActiveStage1 : [(iChmMgrStat != 0) && (iChmMgrStat != 2720)...
          |  &&hasChanged(iChmMgrStat)]
          | {iSendCout = 0;}
      SendAgain -> ActiveStage1 : [tickCount >= ChmReqIntlCnt]
      ActiveStage2 -> ActiveStage1 [order 3] : [((iChmMgrStat != 0) && (iChmMgrStat != 2720))...
          | &&(tickCount >= ChmReqIntlCnt)]
      ActiveStage1 -> ActiveStage2 : [after(ChmReqDurmCnt,tick)]
      ActiveStage2 -> SendAgain [order 2] : [(iChmMgrStat != 0) && (iChmMgrStat != 2720)...
          |  &&hasChanged(iChmMgrStat)]
      ActiveStage2 -> CheckStat.Active.Idle [order 1] : [iSendCout >= 4]
    (default) -> CheckStat.Idle
    CheckStat.Idle -> Active : [((iChmMgrStat != 0) && (iChmMgrStat != 2720))]
  state Idle
    state NoActive
      en:
      oChime = EventSts1.EventSts_NoAct;
      iSendCout = 0;
    state Cancel
      en:
      oChime =  EventSts1.EventSts_CancleChime;
    (default) -> NoActive
    Cancel -> NoActive : //[after(2,tick)]
        | [after(25,tick)]
  note: /*ChmReqDurmTm/10 = 20*/
  note: $0=NO_ACTION; $1=ACTIVE; $2=CANCEL_CHIME
  note: /*KeSMS_u_ChmReqIntlTm/10ms = 5*/
  (default) -> Init
  Init -> Idle
  Idle -> CheckStat : [iChimActive]
  CheckStat -> Cancel : [after(iChimeTm,tick)]
  data: iChmMgrStat input; iChimActive input boolean; iChimeTm input; oChime output Enum: EventSts1; tickCount local uint8 size=1; iKeSMSuChmReqDurmTm input uint8; iKeSMSuChmReqIntlTm input uint8; ChmReqDurmCnt local uint8 size=1; ChmReqIntlCnt local uint8 size=1; iSendCout local uint8 size=1

== stateflow chart ChimeIndicatorOutput/ChimeIndicatorOutputRunnable_sys/Subsystem/SRSIndicator/Subsystem/Chart ==
  (default) -> (junction 6) : {index_i = 1;}
  (junction 6) -> (junction 8) [order 1] : [index_i  <= len]
  (junction 10) -> (junction 6) [order 2] : {index_i++;}
  (junction 6) -> (junction 15) [order 2] : {index_o = 0;}
  (junction 8) -> (junction 10)
  (junction 10) -> (junction 13) [order 1] : [PosArray1[index_i] == idata]
  (junction 13) -> (junction 17) : {index_o = index_i;}
  (junction 17) -> (junction 15)
  (junction 15) -> (junction 22)
  data: PosArray1 input uint8 size=33; len input uint8; idata input uint8; index_i local uint8; index_o output uint8
